simulink model "a1bd1"  (R2020a)
settings: Solver=ode15s  StartTime=0.0  StopTime=10.0  RelTol=1e-3
settings Model: Creator=mumun  LastModifiedBy=mumun
settings SolverCC: ZeroCrossAlgorithm=Adaptive
settings DebuggingCC: IgnoredZcDiagnostic=none

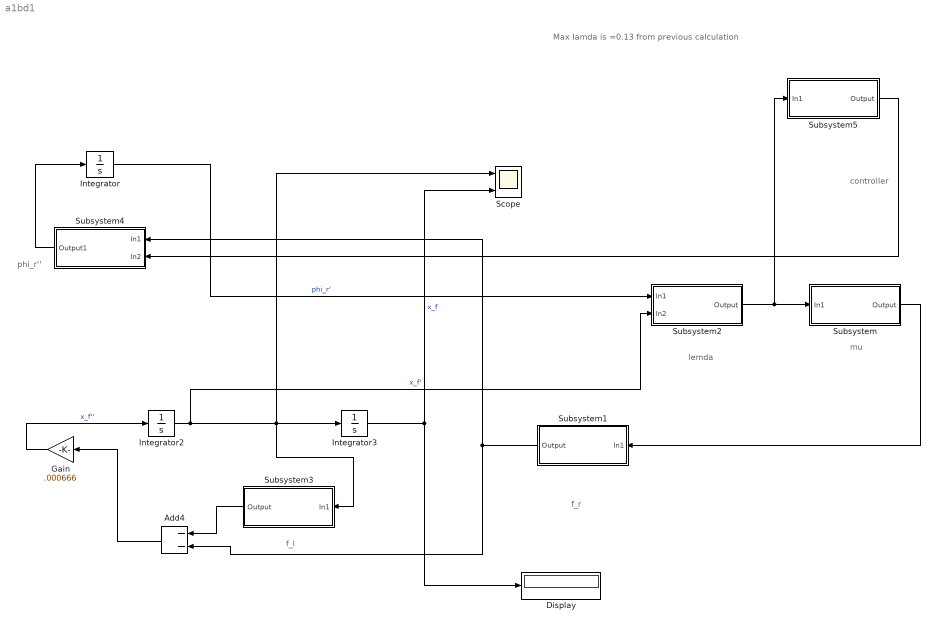
== system a1bd1 ==
  note: Max lamda is =0.13 from previous calculation
  note: phi_r''
  note: controller
  note: f_l
  note: f_r
  note: lemda
  note: mu
  Add4 : Sum  Inputs=--
  Display : Display
  Gain : Gain  Gain=.000666
  Integrator : Integrator  LimitOutput=on  LowerSaturationLimit=0
  Integrator2 : Integrator  InitialCondition=30  LimitOutput=on  LowerSaturationLimit=0
  Integrator3 : Integrator
  Scope : Scope  NumInputPorts=2
  Subsystem : Subsystem
  Subsystem1 : Subsystem
  Subsystem2 : Subsystem
  Subsystem3 : Subsystem
  Subsystem4 : Subsystem
  Subsystem5 : Subsystem
  wires:
  Integrator2/1 -> Subsystem2/2(In2), Integrator3/1, Scope/1, Subsystem3/1(In1)  "x_f'"
  Gain/1 -> Integrator2/1  "x_f''"
  Add4/1 -> Gain/1
  Subsystem/1(Output) -> Subsystem1/1(In1)
  Subsystem1/1(Output) -> Subsystem4/1(In1), Add4/2
  Subsystem3/1(Output) -> Add4/1
  Subsystem4/1(Output1) -> Integrator/1
  Integrator3/1 -> Display/1, Scope/2  "x_f"
  Integrator/1 -> Subsystem2/1(In1)  "phi_r'"
  Subsystem2/1(Output) -> Subsystem5/1(In1), Subsystem/1(In1)
  Subsystem5/1(Output) -> Subsystem4/2(In2)

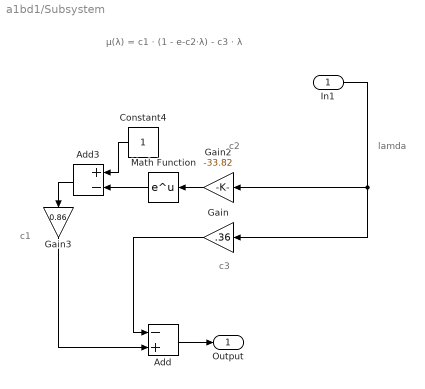
== system a1bd1/Subsystem ==
  note: lamda
  note: c2
  note: c3
  note: c1
  note: µ(λ) = c1 · (1 - e-c2·λ) - c3 · λ
  In1 : Inport
  Add : Sum  Inputs=-+
  Add3 : Sum  Inputs=+-
  Constant4 : Constant
  Gain : Gain  Gain=.36
  Gain2 : Gain  Gain=-33.82
  Gain3 : Gain  Gain=0.86
  Math Function : Math  SaturateOnIntegerOverflow=on
  Output : Outport
  wires:
  Add3/1 -> Gain3/1
  Math Function/1 -> Add3/2
  Constant4/1 -> Add3/1
  Gain2/1 -> Math Function/1
  In1/1 -> Gain/1, Gain2/1
  Gain/1 -> Add/1
  Gain3/1 -> Add/2
  Add/1 -> Output/1

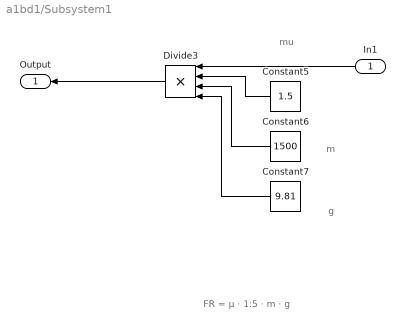
== system a1bd1/Subsystem1 ==
  note: mu
  note: g
  note: m
  note: FR = µ · 1:5 · m · g
  In1 : Inport
  Constant5 : Constant  Value=1.5
  Constant6 : Constant  Value=1500
  Constant7 : Constant  Value=9.81
  Divide3 : Product  Inputs=****
  Output : Outport
  wires:
  Constant6/1 -> Divide3/3
  In1/1 -> Divide3/1
  Constant5/1 -> Divide3/2
  Constant7/1 -> Divide3/4
  Divide3/1 -> Output/1

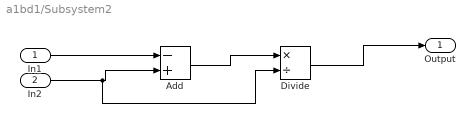
== system a1bd1/Subsystem2 ==
  In1 : Inport
  In2 : Inport  Port=2
  Add : Sum  Inputs=-+
  Divide : Product  Inputs=*/
  Output : Outport
  wires:
  In1/1 -> Add/1
  In2/1 -> Divide/2, Add/2
  Add/1 -> Divide/1
  Divide/1 -> Output/1

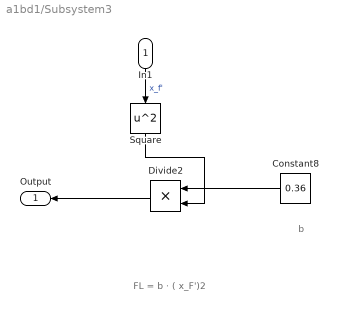
== system a1bd1/Subsystem3 ==
  note: b
  note: FL = b · ( x_F')2
  In1 : Inport
  Constant8 : Constant  Value=0.36
  Divide2 : Product  Inputs=**
  Square : Math  Operator=square  SaturateOnIntegerOverflow=on
  Output : Outport
  wires:
  In1/1 -> Square/1  "x_f'"
  Divide2/1 -> Output/1
  Square/1 -> Divide2/2
  Constant8/1 -> Divide2/1

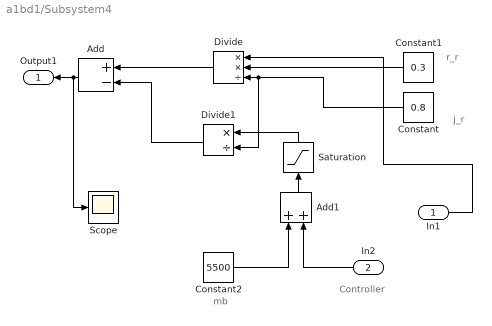
== system a1bd1/Subsystem4 ==
  note: Controller
  note: mb
  note: r_r
  note: j_r
  In1 : Inport
  In2 : Inport  Port=2
  Add : Sum  Inputs=+-
  Add1 : Sum
  Constant : Constant  Value=0.8
  Constant1 : Constant  Value=0.3
  Constant2 : Constant  Value=5500
  Divide : Product  Inputs=**/
  Divide1 : Product  Inputs=*/
  Saturation : Saturate  UpperLimit=inf  LowerLimit=-inf
  Scope : Scope
  Output1 : Outport
  wires:
  Divide/1 -> Add/1
  Divide1/1 -> Add/2
  Constant/1 -> Divide1/2, Divide/3
  Constant1/1 -> Divide/2
  Add/1 -> Scope/1, Output1/1
  In1/1 -> Divide/1
  Constant2/1 -> Add1/1
  In2/1 -> Add1/2
  Add1/1 -> Saturation/1
  Saturation/1 -> Divide1/1

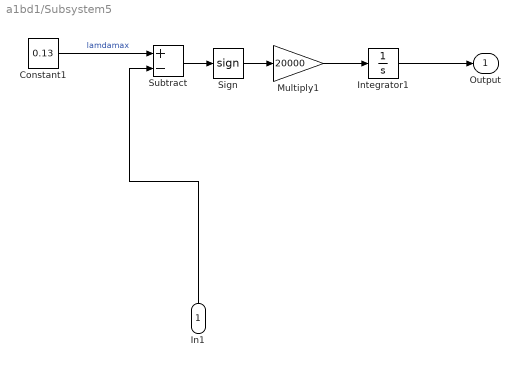
== system a1bd1/Subsystem5 ==
  In1 : Inport
  Constant1 : Constant  Value=0.13
  Integrator1 : Integrator  LimitOutput=on  UpperSaturationLimit=20000  LowerSaturationLimit=-20000
  Multiply1 : Gain  Gain=20000
  Sign : Signum
  Subtract : Sum  Inputs=+-
  Output : Outport
  wires:
  Constant1/1 -> Subtract/1  "lamdamax"
  In1/1 -> Subtract/2
  Subtract/1 -> Sign/1
  Multiply1/1 -> Integrator1/1
  Sign/1 -> Multiply1/1
  Integrator1/1 -> Output/1
